simulink model "cart_pendulum_compact"  (R2020b)
settings: Solver=VariableStepAuto  StartTime=0.0  StopTime=10.0  RelTol=1e-3
values from neighbouring files (symbols this model uses):
  control = ss(acontrol,bcontrol,ccontrol,dcontrol,linmod_k.Ts)    [get_controller.m]    (also in main_cart_pendulum_dlqr.m = get_controller(modelk,ycontrol,add_states,lstates,kobs))
  maxforce = 50    [main_cart_pendulum_dlqr.m]
  setpoint = 0.5    [main_cart_pendulum_dlqr.m]
  x0 = [0; deg2rad(60); 0; 0]    [main_cart_pendulum_dlqr.m]
undefined symbols (not defined in the file or in its folder): ubar, xbar
libraries: cstblocks x1
settings Model: Creator=Kingdel  LastModifiedBy=Usuario

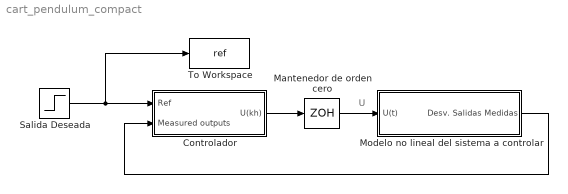
== system cart_pendulum_compact ==
  note: U
  Controlador : Subsystem
  Mantenedor de orden cero : ZeroOrderHold  SampleTime=control.Ts
  Modelo no lineal del sistema a controlar : Subsystem
  Salida Deseada : Step  Time=0  After=setpoint  SampleTime=control.Ts
  To Workspace : ToWorkspace  VariableName=ref  SaveFormat=Structure With Time  SampleTime=control.Ts
  wires:
  Salida Deseada/1 -> Controlador/1(Ref), To Workspace/1
  Mantenedor de orden cero/1 -> Modelo no lineal del sistema a controlar/1(U(t))
  Controlador/1(U(kh)) -> Mantenedor de orden cero/1
  Modelo no lineal del sistema a controlar/1(Desv. Salidas Medidas) -> Controlador/2("Measured outputs ")

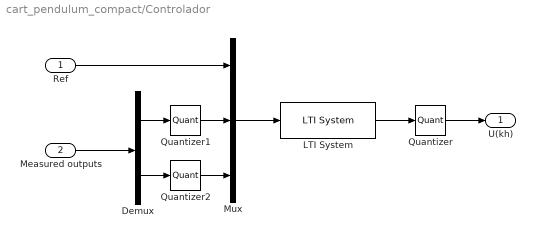
== system cart_pendulum_compact/Controlador ==
  Ref : Inport
  "Measured outputs " : Inport  Port=2
  Demux : Demux  Outputs=2
  LTI System : cstblocks/LTI System  sys=control  IC=[]
  Mux : Mux  Inputs=3
  Quantizer : Quantizer  QuantizationInterval=qforce
  Quantizer1 : Quantizer  QuantizationInterval=qposition
  Quantizer2 : Quantizer  QuantizationInterval=qangle
  U(kh) : Outport
  wires:
  Ref/1 -> Mux/1
  LTI System/1 -> Quantizer/1
  Quantizer/1 -> U(kh)/1
  "Measured outputs "/1 -> Demux/1
  Mux/1 -> LTI System/1
  Quantizer1/1 -> Mux/2
  Demux/1 -> Quantizer1/1
  Quantizer2/1 -> Mux/3
  Demux/2 -> Quantizer2/1

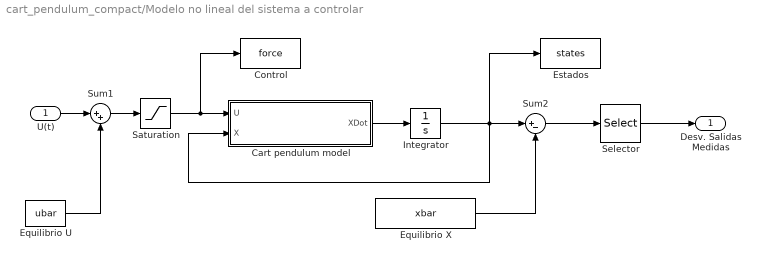
== system cart_pendulum_compact/Modelo no lineal del sistema a controlar ==
  U(t) : Inport
  Cart pendulum model : MATLAB Function  TreatAsAtomicUnit=on
  Control : ToWorkspace  VariableName=force  SaveFormat=Structure With Time  SampleTime=control.Ts
  Equilibrio U : Constant  Value=ubar
  Equilibrio X : Constant  Value=xbar
  Estados : ToWorkspace  VariableName=states  SaveFormat=Structure With Time  SampleTime=control.Ts
  Integrator : Integrator  InitialCondition=x0
  Saturation : Saturate  UpperLimit=maxforce  LowerLimit=-maxforce
  Selector : Selector  InputPortWidth=4  IndexOptions=Index vector (dialog)  Indices=[1 2]  OutputSizes=1
  Sum1 : Sum  Inputs=|++
  Sum2 : Sum  Inputs=|+-
  Desv. Salidas Medidas : Outport  VectorParamsAs1DForOutWhenUnconnected=off
  wires:
  Cart pendulum model/1(XDot) -> Integrator/1
  Integrator/1 -> Cart pendulum model/2(X), Sum2/1, Estados/1
  Equilibrio X/1 -> Sum2/2
  Equilibrio U/1 -> Sum1/2
  U(t)/1 -> Sum1/1
  Sum2/1 -> Selector/1
  Selector/1 -> Desv. Salidas Medidas/1
  Saturation/1 -> Control/1, Cart pendulum model/1(U)
  Sum1/1 -> Saturation/1

== matlab function cart_pendulum_compact/Modelo no lineal del sistema a controlar/Cart pendulum model ==
  data: U input; XDot output; X input
function XDot = cart_pendulum_model(U,X)
%#codegen
% Constants of the model
[M,m,J,L,a,g] = deal(1,0.1,0.025,0.5,0.5,9.807);                      
[X1,X2,X3,X4] = deal(X(1),X(2),X(3),X(4));

% Inertia matrix
D           = [M+m,-m*a*L*sin(X2);-m*a*L*sin(X2),m*a^2*L^2+J];

% Coriolis and centrifugal forces
H           = [-m*a*L*cos(X2)*X4^2; +m*a*L*g*cos(X2)];

% Impact detection
F           = impact_force(M+m,X1,X3);
U           = U + F;

% Generalized effort
E           = [U; 0];

% State space model
% x1 = x, x2 = theta, x3 = xdot, x4 = thetadot
XDot        = [X3; X4; D\(E-H)];
end

% Force for left impact
function F  = impact_force(Mass,Pos,Vel)
% Settling time
Ts          = 0.01;
% Damping 
Xi          = 0.707;
% Natural frequency
Wn          = 4/(Ts*Xi);
% Spring constant
Kp          = Mass*Wn^2;
% Damper constant
Kv          = 2*Mass*Xi*Wn;
F           = 0;
% Impact force
Limit       = 1.7;
if Pos < -Limit && Vel < 0
    F       = -Kp*(Pos+Limit) -Kv*Vel;
elseif Pos > Limit && Vel > 0
    F       = -Kp*(Pos-Limit) -Kv*Vel;
end
end
